simulink model "Open_loop_Response_ODBP"  (R2020a)
settings: Solver=VariableStepAuto  StartTime=0.0  StopTime=10  RelTol=1e-3
values from neighbouring files (symbols this model uses):
  d = 0.03    [Root_Locus.m]
  g = -9.8    [Root_Locus.m]
  J = 9.99e-6    (= 9.99e-06)    [Root_Locus.m]
  L = 1.0    (= 1)    [Root_Locus.m]
  m = 0.111    [Root_Locus.m]
  R = 0.015    [Root_Locus.m]
settings Model: Creator=jgrou  LastModifiedBy=jgrou

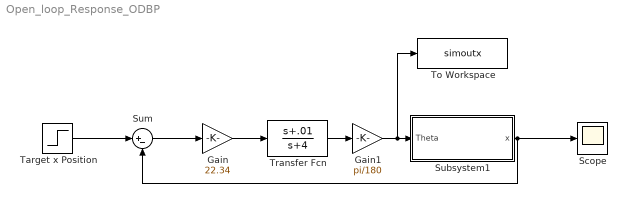
== system Open_loop_Response_ODBP ==
  Gain : Gain  Gain=22.34
  Gain1 : Gain  Gain=pi/180
  Scope : Scope
  Subsystem1 : Subsystem
  Sum : Sum  Inputs=|+-
  Target x Position : Step  Time=0  SampleTime=0
  To Workspace : ToWorkspace  VariableName=simoutx  SaveFormat=Timeseries  SampleTime=-1
  Transfer Fcn : TransferFcn  Numerator=[1 .01]  Denominator=[1 4]
  wires:
  Subsystem1/1(x) -> Sum/2, Scope/1
  Target x Position/1 -> Sum/1
  Sum/1 -> Gain/1
  Gain/1 -> Transfer Fcn/1
  Gain1/1 -> To Workspace/1, Subsystem1/1(Theta)
  Transfer Fcn/1 -> Gain1/1

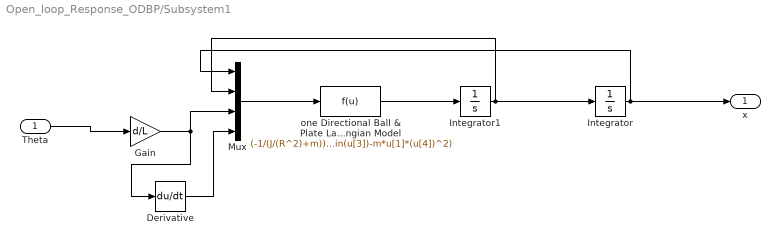
== system Open_loop_Response_ODBP/Subsystem1 ==
  Theta : Inport
  Derivative : Derivative
  Gain : Gain  Gain=d/L
  Integrator : Integrator
  Integrator1 : Integrator
  Mux : Mux
  one Directional Ball & Plate Lagrangian Model : Fcn  Expr=(-1/(J/(R^2)+m))*(m*g*sin(u[3])-m*u[1]*(u[4])^2)
  x : Outport
  wires:
  Theta/1 -> Gain/1
  Gain/1 -> Mux/3, Derivative/1
  one Directional Ball & Plate Lagrangian Model/1 -> Integrator1/1
  Derivative/1 -> Mux/4
  Mux/1 -> one Directional Ball & Plate Lagrangian Model/1
  Integrator/1 -> Mux/1, x/1
  Integrator1/1 -> Mux/2, Integrator/1
